simulink model "ValidacionAlgebraicoFJHON"  (R2021b)
settings: Solver=VariableStepAuto  StartTime=0.0  StopTime=5  RelTol=1e-3
undefined symbols (not defined in the file or in its folder): F
libraries: cstblocks x2
settings Model: Creator=axelt  LastModifiedBy=parra
settings DebuggingCC: UnconnectedInputMsg=none  UnconnectedOutputMsg=none  UnconnectedLineMsg=none
settings ModelReferenceCC: EnableRefExpFcnMdlSchedulingChecks=off
settings RTWCC: DLArmComputeVersion=20.02.1

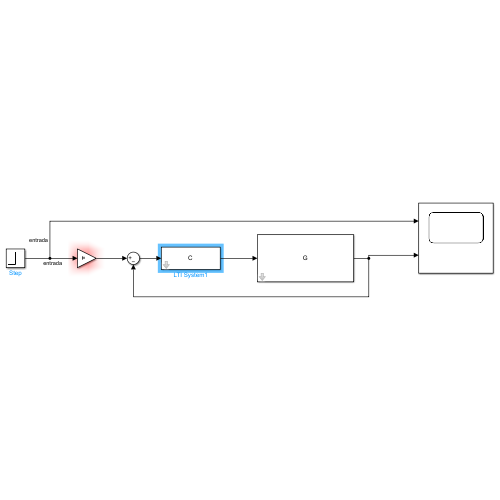
[thumbnail: Simulink's stored preview of the top-level diagram]
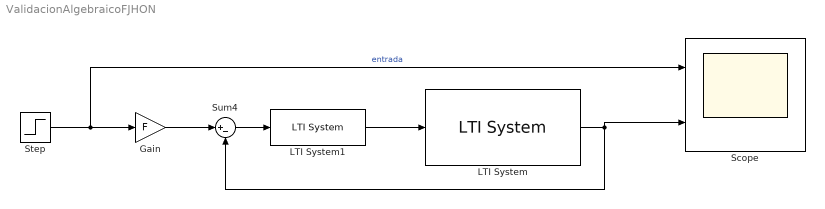
== system ValidacionAlgebraicoFJHON ==
  Gain : Gain  Gain=F
  LTI System : cstblocks/LTI System  sys=G  IC=[]
  LTI System1 : cstblocks/LTI System  sys=C  IC=[]
  Scope : Scope  NumInputPorts=2
  Step : Step  Time=20  Before=0.5  SampleTime=0.01
  Sum4 : Sum  Inputs=|+-
  wires:
  Step/1 -> Gain/1, Scope/1  "entrada"
  Sum4/1 -> LTI System1/1
  LTI System/1 -> Scope/2, Sum4/2
  Gain/1 -> Sum4/1
  LTI System1/1 -> LTI System/1
